simulink model "gm_CustArchitecture_vnl"  (R2020a)
settings: Solver=FixedStepDiscrete  StartTime=0.0  StopTime=840000  RelTol=1e-3
libraries: simulink x92, hdlsllib x56, IIT_Genoa_Intan_HDL_blocks x7
(part 1 of 3)
settings Model: FPTRunName=FPA_Reference  PacingRate=40  Creator=BuccelliLab  LastModifiedBy=diflo
settings SolverCC: AutoInsertRateTranBlk=on  MinimalZcImpactIntegration=on
settings DataIOCC: LimitDataPoints=on  SaveOutput=off  SaveTime=off  ReturnWorkspaceOutputs=off
settings OptimizationCC: BlockReduction=off  ConditionallyExecuteInputs=off  DefaultParameterBehavior=Inlined  LifeSpan=inf
settings DebuggingCC: SignalRangeChecking=warning  ReadBeforeWriteMsg=DisableAll  WriteAfterWriteMsg=DisableAll  WriteAfterReadMsg=DisableAll  AlgebraicLoopMsg=error  InheritedTsInSrcMsg=none  MultiTaskDSMMsg=none  SingleTaskRateTransMsg=error  ParameterDowncastMsg=warning  ParameterOverflowMsg=warning  AllowSymbolicDim=off  StrictBusMsg=ErrorOnBusTreatedAsVector  SFUnexpectedBacktrackingDiag=warning  SFNoUnconditionalDefaultTransitionDiag=warning  SFExecutionAtInitializationDiag=none  ArithmeticOperatorsInVariantConditions=warning
settings HardwareCC: ProdBitPerPointer=32  ProdBitPerSizeT=32  ProdBitPerPtrDiffT=32  ProdLargestAtomicFloat=None  ProdIntDivRoundTo=Undefined  ProdEndianess=Unspecified  ProdWordSize=32  ProdHWDeviceType=ASIC/FPGA->ASIC/FPGA  TargetBitPerPointer=64  TargetBitPerSizeT=64  TargetBitPerPtrDiffT=64  TargetLongLongMode=on  TargetIntDivRoundTo=Zero  TargetEndianess=LittleEndian  TargetWordSize=64  TargetHWDeviceType=Custom Processor->MATLAB Host Computer  ProdEqTarget=off
settings ModelReferenceCC: UpdateModelReferenceTargets=IfOutOfDate
settings SFSimCC: SFSimEcho=off  SimUseLocalCustomCode=off  CustomCodeUndefinedFunction=UseInterfaceOnly
settings RTWCC: RTWUseLocalCustomCode=off
settings CodeAppCC: StateflowObjectComments=on
settings GRTTargetCC: TargetLangStandard=C89/C90 (ANSI)
settings ConfigComp: CovScope=ReferencedModels  CovMetricSettings=dw  CovHtmlReporting=on  CovSaveCumulativeToWorkspaceVar=on  CovSaveSingleToWorkspaceVar=on  CovExternalEMLEnable=off  CovSFcnEnable=off

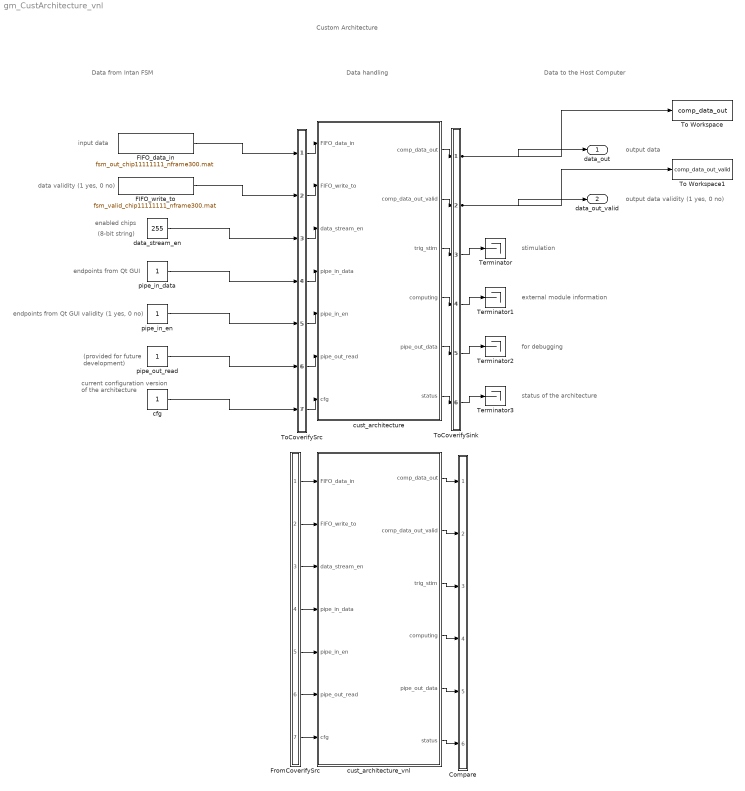
== system gm_CustArchitecture_vnl ==
  note: Data handling
  note: Custom Architecture
  note: output data validity (1 yes, 0 no)
  note: endpoints from Qt GUI
  note: (8-bit string)
  note: enabled chips
  note: data validity (1 yes, 0 no)
  note: input data
  note: endpoints from Qt GUI validity (1 yes, 0 no)
  note: (provided for future
      | development)
  note: current configuration
      | version of the
      | architecture
  note: output data
  note: Data to the Host Computer
  note: stimulation
  note: external module information
  note: for debugging
  note: status of the architecture
  note: Data from Intan FSM
  Compare : Subsystem
      mask Display: disp('')
  FIFO_data_in : FromFile  FileName=fsm_out_chip11111111_nframe300.mat  OutDataTypeStr=uint16  SampleTime=1  ExtrapolationBeforeFirstDataPoint=Hold first value  InterpolationWithinTimeRange=Zero order hold  ExtrapolationAfterLastDataPoint=Hold last value
  FIFO_write_to : FromFile  FileName=fsm_valid_chip11111111_nframe300.mat  OutDataTypeStr=boolean  SampleTime=1
  FromCoverifySrc : Subsystem
      mask Display: disp('')
  Terminator{,1..3} (4 alike) : Terminator
  To Workspace : ToWorkspace  VariableName=comp_data_out  SaveFormat=Timeseries  SampleTime=-1
  To Workspace1 : ToWorkspace  VariableName=comp_data_out_valid  SaveFormat=Timeseries  SampleTime=-1
  ToCoverifySink : Subsystem
      mask Display: disp('')
  ToCoverifySrc : Subsystem
      mask Display: disp('')
  cfg : Constant  OutDataTypeStr=uint16  SampleTime=-1
  cust_architecture : Subsystem
  cust_architecture_vnl : Subsystem
  data_stream_en : Constant  Value=255  OutDataTypeStr=uint8  SampleTime=-1
  pipe_in_data : Constant  OutDataTypeStr=uint16  SampleTime=-1
  pipe_in_en : Constant  OutDataTypeStr=boolean  SampleTime=-1
  pipe_out_read : Constant  OutDataTypeStr=boolean  SampleTime=-1
  data_out : Outport  VectorParamsAs1DForOutWhenUnconnected=off
  data_out_valid : Outport  Port=2  VectorParamsAs1DForOutWhenUnconnected=off
  wires:
  ToCoverifySrc/1(out1) -> cust_architecture/1(FIFO_data_in)
  ToCoverifySrc/2(out2) -> cust_architecture/2(FIFO_write_to)
  ToCoverifySrc/3(out3) -> cust_architecture/3(data_stream_en)
  ToCoverifySrc/4(out4) -> cust_architecture/4(pipe_in_data)
  ToCoverifySrc/5(out5) -> cust_architecture/5(pipe_in_en)
  ToCoverifySrc/6(out6) -> cust_architecture/6(pipe_out_read)
  ToCoverifySrc/7(out7) -> cust_architecture/7(cfg)
  cust_architecture/1(comp_data_out) -> ToCoverifySink/1(in1)
  cust_architecture/2(comp_data_out_valid) -> ToCoverifySink/2(in2)
  cust_architecture/3(trig_stim) -> ToCoverifySink/3(in3)
  cust_architecture/4(computing) -> ToCoverifySink/4(in4)
  cust_architecture/5(pipe_out_data) -> ToCoverifySink/5(in5)
  cust_architecture/6(status) -> ToCoverifySink/6(in6)
  FIFO_data_in/1 -> ToCoverifySrc/1(in1)
  FIFO_write_to/1 -> ToCoverifySrc/2(in2)
  data_stream_en/1 -> ToCoverifySrc/3(in3)
  pipe_in_data/1 -> ToCoverifySrc/4(in4)
  pipe_in_en/1 -> ToCoverifySrc/5(in5)
  pipe_out_read/1 -> ToCoverifySrc/6(in6)
  cfg/1 -> ToCoverifySrc/7(in7)
  ToCoverifySink/1(out1) -> data_out/1, To Workspace/1
  ToCoverifySink/2(out2) -> data_out_valid/1, To Workspace1/1
  ToCoverifySink/3(out3) -> Terminator/1
  ToCoverifySink/4(out4) -> Terminator1/1
  ToCoverifySink/5(out5) -> Terminator2/1
  ToCoverifySink/6(out6) -> Terminator3/1
  FromCoverifySrc/1(out1) -> cust_architecture_vnl/1(FIFO_data_in)
  FromCoverifySrc/2(out2) -> cust_architecture_vnl/2(FIFO_write_to)
  FromCoverifySrc/3(out3) -> cust_architecture_vnl/3(data_stream_en)
  FromCoverifySrc/4(out4) -> cust_architecture_vnl/4(pipe_in_data)
  FromCoverifySrc/5(out5) -> cust_architecture_vnl/5(pipe_in_en)
  FromCoverifySrc/6(out6) -> cust_architecture_vnl/6(pipe_out_read)
  FromCoverifySrc/7(out7) -> cust_architecture_vnl/7(cfg)
  cust_architecture_vnl/1(comp_data_out) -> Compare/1(in1)
  cust_architecture_vnl/2(comp_data_out_valid) -> Compare/2(in2)
  cust_architecture_vnl/3(trig_stim) -> Compare/3(in3)
  cust_architecture_vnl/4(computing) -> Compare/4(in4)
  cust_architecture_vnl/5(pipe_out_data) -> Compare/5(in5)
  cust_architecture_vnl/6(status) -> Compare/6(in6)

== system gm_CustArchitecture_vnl/Compare ==
  in1 : Inport
  in2 : Inport  Port=2
  in3 : Inport  Port=3
  in4 : Inport  Port=4
  in5 : Inport  Port=5
  in6 : Inport  Port=6
  Assert_comp_data_out : Subsystem
  Assert_comp_data_out_valid : Subsystem
  Assert_computing : Subsystem
  Assert_pipe_out_data : Subsystem
  Assert_status : Subsystem
  Assert_trig_stim : Subsystem
  CleanupScopes : Subsystem
      settings: OpenFcn=|
      | blkName = gcb; %self block
      | idx = regexp(blkName, '/CleanupScopes$', 'once');
      | blkParent = blkName(1:idx-1);
      | blks=find_system(blkParent, 'LookUnderMasks', 'all','blocktype', 'Scope');
      | for itr = 1:length(blks)
      | 	 hScopeCfg = get_param(blks{itr},'ScopeConfiguration');
      | 	 hScopeCfg.Visible = ~ hScopeCfg.Visible;
      | end
      | drawnow;
      mask Display: fprintf(message('hdlcoder:cosim:vnl_dblclick').getString());
  Enable : Subsystem
      settings: OpenFcn=|
      | blkName = gcb;
      | idx = regexp(blkName, '/Enable$', 'once');
      | blkParent = blkName(1:idx-1);
      | blks=find_system(blkParent, 'LookUnderMasks', 'all','blocktype', 'Assertion');
      | e = get_param(blks{1}, 'Enabled');
      | if strcmp(e, 'on'), f= 'off';, else, f = 'on';, end
      | for ii=1:length(blks), set_param(blks{ii}, 'Enabled', f);, end
      | set_param(gcb, 'MaskDisplay',['fprintf(message(''hdlcoder:cosim:vnl_dblclick_assertions'',','''',upper(e),'''',').getString())']);
      mask Display: fprintf(message('hdlcoder:cosim:vnl_dblclick_assertions','OFF').getString());
  wires:
  in1/1 -> Assert_comp_data_out/1(cosim)
  [out1] -> Assert_comp_data_out/2(dut)
  in2/1 -> Assert_comp_data_out_valid/1(cosim)
  [out2] -> Assert_comp_data_out_valid/2(dut)
  in3/1 -> Assert_trig_stim/1(cosim)
  [out3] -> Assert_trig_stim/2(dut)
  in4/1 -> Assert_computing/1(cosim)
  [out4] -> Assert_computing/2(dut)
  in5/1 -> Assert_pipe_out_data/1(cosim)
  [out5] -> Assert_pipe_out_data/2(dut)
  in6/1 -> Assert_status/1(cosim)
  [out6] -> Assert_status/2(dut)

== system gm_CustArchitecture_vnl/FromCoverifySrc ==
  out1 : Outport
  out2 : Outport  Port=2
  out3 : Outport  Port=3
  out4 : Outport  Port=4
  out5 : Outport  Port=5
  out6 : Outport  Port=6
  out7 : Outport  Port=7
  wires:
  [in1] -> out1/1
  [in2] -> out2/1
  [in3] -> out3/1
  [in4] -> out4/1
  [in5] -> out5/1
  [in6] -> out6/1
  [in7] -> out7/1

== system gm_CustArchitecture_vnl/ToCoverifySink ==
  in1 : Inport
  in2 : Inport  Port=2
  in3 : Inport  Port=3
  in4 : Inport  Port=4
  in5 : Inport  Port=5
  in6 : Inport  Port=6
  out1 : Outport
  out2 : Outport  Port=2
  out3 : Outport  Port=3
  out4 : Outport  Port=4
  out5 : Outport  Port=5
  out6 : Outport  Port=6
  tag scope: out1=global, out2=global, out3=global, out4=global, out5=global, out6=global
  wires:
  in1/1 -> out1/1, [out1]
  in2/1 -> out2/1, [out2]
  in3/1 -> out3/1, [out3]
  in4/1 -> out4/1, [out4]
  in5/1 -> out5/1, [out5]
  in6/1 -> out6/1, [out6]

== system gm_CustArchitecture_vnl/ToCoverifySrc ==
  in1 : Inport
  in2 : Inport  Port=2
  in3 : Inport  Port=3
  in4 : Inport  Port=4
  in5 : Inport  Port=5
  in6 : Inport  Port=6
  in7 : Inport  Port=7
  out1 : Outport
  out2 : Outport  Port=2
  out3 : Outport  Port=3
  out4 : Outport  Port=4
  out5 : Outport  Port=5
  out6 : Outport  Port=6
  out7 : Outport  Port=7
  tag scope: in1=global, in2=global, in3=global, in4=global, in5=global, in6=global, in7=global
  wires:
  in1/1 -> out1/1, [in1]
  in2/1 -> out2/1, [in2]
  in3/1 -> out3/1, [in3]
  in4/1 -> out4/1, [in4]
  in5/1 -> out5/1, [in5]
  in6/1 -> out6/1, [in6]
  in7/1 -> out7/1, [in7]

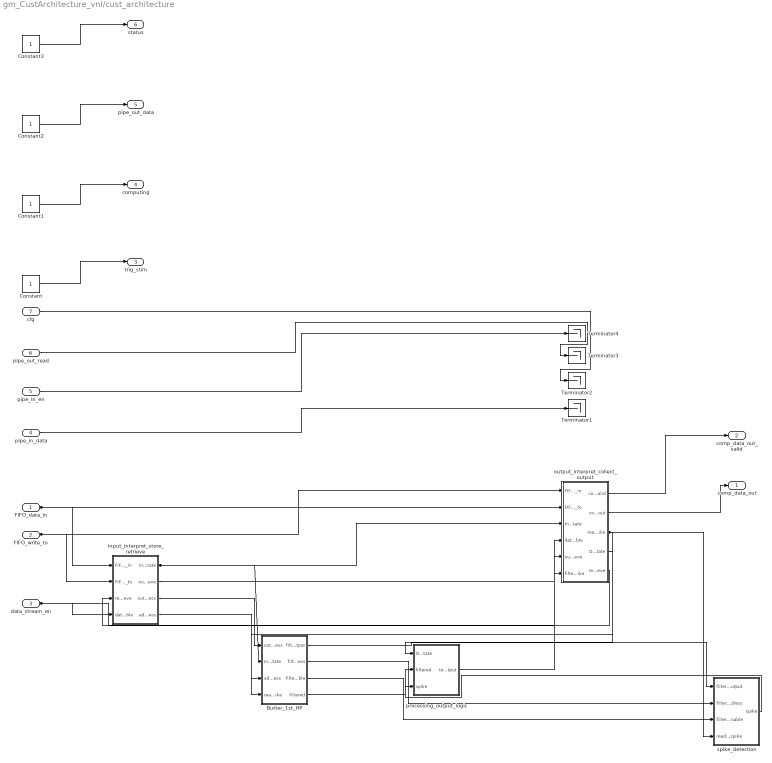
== system gm_CustArchitecture_vnl/cust_architecture ==
  FIFO_data_in : Inport  OutDataTypeStr=uint16  PortDimensions=1  SampleTime=1
  FIFO_write_to : Inport  Port=2  OutDataTypeStr=boolean  PortDimensions=1  SampleTime=1
  data_stream_en : Inport  Port=3  OutDataTypeStr=uint8  PortDimensions=1  SampleTime=1
  pipe_in_data : Inport  Port=4  OutDataTypeStr=uint16  PortDimensions=1  SampleTime=1
  pipe_in_en : Inport  Port=5  OutDataTypeStr=boolean  PortDimensions=1  SampleTime=1
  pipe_out_read : Inport  Port=6  OutDataTypeStr=boolean  PortDimensions=1  SampleTime=1
  cfg : Inport  Port=7  OutDataTypeStr=uint16  PortDimensions=1  SampleTime=1
  Butter_1st_HP : Subsystem  mask{s1=double(0.9695312529087462), a21=double(-0.9390625058174924)}
      mask Display:
      | color('white'); port_label('input',1,'output_data_to_process')
      | color('white'); port_label('input',2,'InputState')
      | color('white'); port_label('input',3,'address_output_data_to_process')
      | color('white'); port_label('input',4,'read_filter_output_or_spike')
      | color('white'); port_label('output',1,'filter_output')
      | color('white'); port_label('output',2,'filter_writing_address')
      | color('white'); port_label('output',3,'filter_writing_enable')
      | color('white'); port_label('output',4,'filtered')
  Constant : Constant  OutDataTypeStr=uint8  SampleTime=1
  Constant1 : Constant  OutDataTypeStr=boolean  SampleTime=1
  Constant2 : Constant  OutDataTypeStr=uint16  SampleTime=1
  Constant3 : Constant  OutDataTypeStr=uint16  SampleTime=1
  Terminator{1..4} (4 alike) : Terminator
  input_interpret_store_retrieve : Subsystem
  output_interpret_collect_output : Subsystem
  processing_output_logic : Subsystem
  spike_detection : Subsystem
  comp_data_out : Outport  VectorParamsAs1DForOutWhenUnconnected=off
  comp_data_out_valid : Outport  Port=2  OutDataTypeStr=boolean  VectorParamsAs1DForOutWhenUnconnected=off
  trig_stim : Outport  Port=3  VectorParamsAs1DForOutWhenUnconnected=off
  computing : Outport  Port=4  VectorParamsAs1DForOutWhenUnconnected=off
  pipe_out_data : Outport  Port=5  VectorParamsAs1DForOutWhenUnconnected=off
  status : Outport  Port=6  VectorParamsAs1DForOutWhenUnconnected=off
  wires:
  spike_detection/1(spike) -> processing_output_logic/3(spike)
  processing_output_logic/1(to_output_interpret_collect_output) -> output_interpret_collect_output/6(filter_output_or_spike)
  output_interpret_collect_output/5(read_output_data_input_interpret_store_retrieve) -> input_interpret_store_retrieve/3(read_output_data_input_interpret_store_retrieve)
  output_interpret_collect_output/4(OutputState) -> processing_output_logic/1(OutputState)
  output_interpret_collect_output/3(read_filter_output_or_spike) -> Butter_1st_HP/4(read_filter_output_or_spike), spike_detection/4(read_filter_output_or_spike)
  output_interpret_collect_output/2(comp_data_out) -> comp_data_out/1
  output_interpret_collect_output/1(comp_data_out_valid) -> comp_data_out_valid/1
  input_interpret_store_retrieve/4(address_output_data_to_process) -> Butter_1st_HP/3(address_output_data_to_process)
  input_interpret_store_retrieve/3(output_data_to_process) -> Butter_1st_HP/1(output_data_to_process)
  input_interpret_store_retrieve/2(output_data_input_interpret_store_retrieve) -> output_interpret_collect_output/5(output_data_input_interpret_store_retrieve)
  input_interpret_store_retrieve/1(InputState) -> output_interpret_collect_output/3(InputState), Butter_1st_HP/2(InputState)
  Constant3/1 -> status/1
  Constant2/1 -> pipe_out_data/1
  Constant1/1 -> computing/1
  Constant/1 -> trig_stim/1
  Butter_1st_HP/4(filtered) -> processing_output_logic/2(filtered)
  Butter_1st_HP/3(filter_writing_enable) -> spike_detection/3(filter_writing_enable)
  Butter_1st_HP/2(filter_writing_address) -> spike_detection/2(filter_writing_address)
  Butter_1st_HP/1(filter_output) -> spike_detection/1(filter_output)
  cfg/1 -> Terminator2/1
  pipe_out_read/1 -> Terminator3/1
  pipe_in_en/1 -> Terminator4/1
  pipe_in_data/1 -> Terminator1/1
  data_stream_en/1 -> input_interpret_store_retrieve/4(data_stream_enable), output_interpret_collect_output/4(data_stream_enable)
  FIFO_write_to/1 -> output_interpret_collect_output/2(FIFO_write_to), input_interpret_store_retrieve/2(FIFO_write_to)
  FIFO_data_in/1 -> output_interpret_collect_output/1(FIFO_data_in), input_interpret_store_retrieve/1(FIFO_data_in)

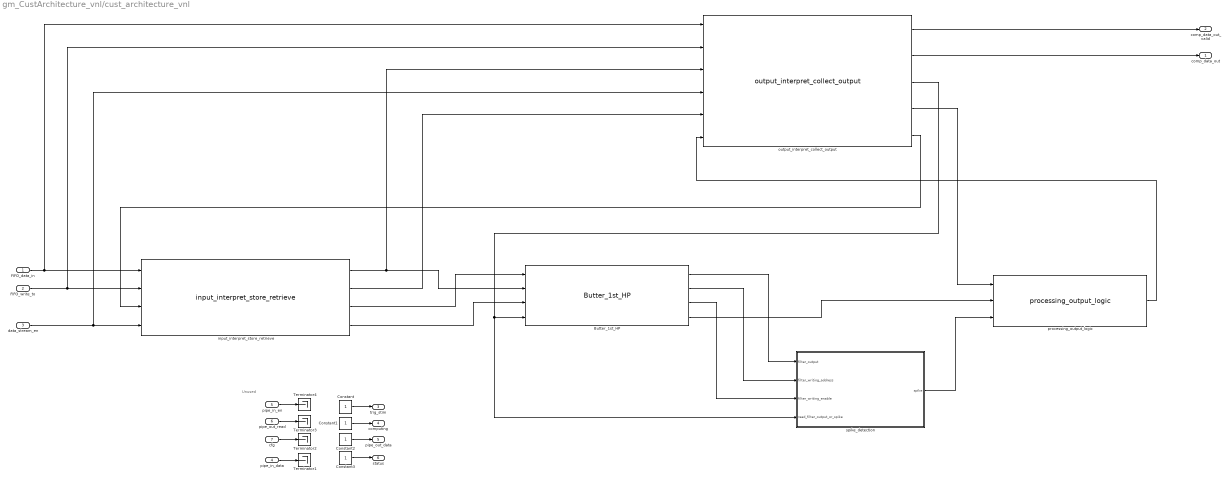
== system gm_CustArchitecture_vnl/cust_architecture_vnl ==
  note: Unused
  FIFO_data_in : Inport
  FIFO_write_to : Inport  Port=2
  data_stream_en : Inport  Port=3
  pipe_in_data : Inport  Port=4
  pipe_in_en : Inport  Port=5
  pipe_out_read : Inport  Port=6
  cfg : Inport  Port=7
  Butter_1st_HP : IIT_Genoa_Intan_HDL_blocks/Filters/Butter_1st_HP  s1=0.969531252908746199  a21=-0.939062505817492399
      settings: SourceProductName=IIT Genoa Intan HDL blocks
  Constant : Constant  OutDataTypeStr=uint8  SampleTime=-1
  Constant1 : Constant  OutDataTypeStr=boolean  SampleTime=-1
  Constant2 : Constant  OutDataTypeStr=uint16  SampleTime=-1
  Constant3 : Constant  OutDataTypeStr=uint16  SampleTime=-1
  Terminator{1..4} (4 alike) : Terminator
  input_interpret_store_retrieve : IIT_Genoa_Intan_HDL_blocks/Encoding//Decoding/input_interpret_store_retrieve
      settings: SourceProductName=IIT Genoa Intan HDL blocks
  output_interpret_collect_output : IIT_Genoa_Intan_HDL_blocks/Encoding//Decoding/output_interpret_collect_output
      settings: SourceProductName=IIT Genoa Intan HDL blocks
  processing_output_logic : IIT_Genoa_Intan_HDL_blocks/Encoding//Decoding/processing_output_logic
      settings: SourceProductName=IIT Genoa Intan HDL blocks
  spike_detection : Subsystem
  comp_data_out : Outport  VectorParamsAs1DForOutWhenUnconnected=off
  comp_data_out_valid : Outport  Port=2  OutDataTypeStr=boolean  VectorParamsAs1DForOutWhenUnconnected=off
  trig_stim : Outport  Port=3  VectorParamsAs1DForOutWhenUnconnected=off
  computing : Outport  Port=4  VectorParamsAs1DForOutWhenUnconnected=off
  pipe_out_data : Outport  Port=5  VectorParamsAs1DForOutWhenUnconnected=off
  status : Outport  Port=6  VectorParamsAs1DForOutWhenUnconnected=off
  wires:
  input_interpret_store_retrieve/4 -> Butter_1st_HP/3
  input_interpret_store_retrieve/3 -> Butter_1st_HP/1
  spike_detection/1(spike) -> processing_output_logic/3
  Butter_1st_HP/3 -> spike_detection/3(filter_writing_enable)
  Butter_1st_HP/2 -> spike_detection/2(filter_writing_address)
  Butter_1st_HP/1 -> spike_detection/1(filter_output)
  processing_output_logic/1 -> output_interpret_collect_output/6
  input_interpret_store_retrieve/1 -> output_interpret_collect_output/3, Butter_1st_HP/2
  input_interpret_store_retrieve/2 -> output_interpret_collect_output/5
  Butter_1st_HP/4 -> processing_output_logic/2
  output_interpret_collect_output/3 -> Butter_1st_HP/4, spike_detection/4(read_filter_output_or_spike)
  output_interpret_collect_output/4 -> processing_output_logic/1
  output_interpret_collect_output/5 -> input_interpret_store_retrieve/3
  output_interpret_collect_output/2 -> comp_data_out/1
  output_interpret_collect_output/1 -> comp_data_out_valid/1
  pipe_in_data/1 -> Terminator1/1
  data_stream_en/1 -> input_interpret_store_retrieve/4, output_interpret_collect_output/4
  FIFO_write_to/1 -> output_interpret_collect_output/2, input_interpret_store_retrieve/2
  FIFO_data_in/1 -> output_interpret_collect_output/1, input_interpret_store_retrieve/1
  pipe_in_en/1 -> Terminator4/1
  pipe_out_read/1 -> Terminator3/1
  cfg/1 -> Terminator2/1
  Constant3/1 -> status/1
  Constant2/1 -> pipe_out_data/1
  Constant1/1 -> computing/1
  Constant/1 -> trig_stim/1

== system gm_CustArchitecture_vnl/Compare/Assert_comp_data_out ==
  cosim : Inport
  dut : Inport  Port=2
  AssertEq : Assertion  StopWhenAssertionFail=off
  Compare To Zero : simulink/Logic and Bit Operations/Compare To Zero  relop===  OutDataTypeStr=boolean
  Relational Operator : RelationalOperator  Operator===  OutDataTypeStr=boolean  RndMeth=Nearest
  compare: comp_data_out : Scope  NumInputPorts=3
  wires:
  Compare To Zero/1 -> compare: comp_data_out/3  "err"
  Relational Operator/1 -> Compare To Zero/1, AssertEq/1
  cosim/1 -> compare: comp_data_out/1, Relational Operator/1  "cosim"
  dut/1 -> compare: comp_data_out/2, Relational Operator/2  "dut ref"

== system gm_CustArchitecture_vnl/Compare/Assert_comp_data_out_valid ==
  cosim : Inport
  dut : Inport  Port=2
  AssertEq : Assertion  StopWhenAssertionFail=off
  Compare To Zero : simulink/Logic and Bit Operations/Compare To Zero  relop===  OutDataTypeStr=boolean
  Relational Operator : RelationalOperator  Operator===  OutDataTypeStr=boolean  RndMeth=Nearest
  compare: comp_data_out_valid : Scope  NumInputPorts=3
  wires:
  Compare To Zero/1 -> compare: comp_data_out_valid/3  "err"
  Relational Operator/1 -> Compare To Zero/1, AssertEq/1
  cosim/1 -> compare: comp_data_out_valid/1, Relational Operator/1  "cosim"
  dut/1 -> compare: comp_data_out_valid/2, Relational Operator/2  "dut ref"

== system gm_CustArchitecture_vnl/Compare/Assert_computing ==
  cosim : Inport
  dut : Inport  Port=2
  AssertEq : Assertion  StopWhenAssertionFail=off
  Compare To Zero : simulink/Logic and Bit Operations/Compare To Zero  relop===  OutDataTypeStr=boolean
  Relational Operator : RelationalOperator  Operator===  OutDataTypeStr=boolean  RndMeth=Nearest
  compare: computing : Scope  NumInputPorts=3
  wires:
  Compare To Zero/1 -> compare: computing/3  "err"
  Relational Operator/1 -> Compare To Zero/1, AssertEq/1
  cosim/1 -> compare: computing/1, Relational Operator/1  "cosim"
  dut/1 -> compare: computing/2, Relational Operator/2  "dut ref"

== system gm_CustArchitecture_vnl/Compare/Assert_pipe_out_data ==
  cosim : Inport
  dut : Inport  Port=2
  AssertEq : Assertion  StopWhenAssertionFail=off
  Compare To Zero : simulink/Logic and Bit Operations/Compare To Zero  relop===  OutDataTypeStr=boolean
  Relational Operator : RelationalOperator  Operator===  OutDataTypeStr=boolean  RndMeth=Nearest
  compare: pipe_out_data : Scope  NumInputPorts=3
  wires:
  Compare To Zero/1 -> compare: pipe_out_data/3  "err"
  Relational Operator/1 -> Compare To Zero/1, AssertEq/1
  cosim/1 -> compare: pipe_out_data/1, Relational Operator/1  "cosim"
  dut/1 -> compare: pipe_out_data/2, Relational Operator/2  "dut ref"

== system gm_CustArchitecture_vnl/Compare/Assert_status ==
  cosim : Inport
  dut : Inport  Port=2
  AssertEq : Assertion  StopWhenAssertionFail=off
  Compare To Zero : simulink/Logic and Bit Operations/Compare To Zero  relop===  OutDataTypeStr=boolean
  Relational Operator : RelationalOperator  Operator===  OutDataTypeStr=boolean  RndMeth=Nearest
  compare: status : Scope  NumInputPorts=3
  wires:
  Compare To Zero/1 -> compare: status/3  "err"
  Relational Operator/1 -> Compare To Zero/1, AssertEq/1
  cosim/1 -> compare: status/1, Relational Operator/1  "cosim"
  dut/1 -> compare: status/2, Relational Operator/2  "dut ref"

== system gm_CustArchitecture_vnl/Compare/Assert_trig_stim ==
  cosim : Inport
  dut : Inport  Port=2
  AssertEq : Assertion  StopWhenAssertionFail=off
  Compare To Zero : simulink/Logic and Bit Operations/Compare To Zero  relop===  OutDataTypeStr=boolean
  Relational Operator : RelationalOperator  Operator===  OutDataTypeStr=boolean  RndMeth=Nearest
  compare: trig_stim : Scope  NumInputPorts=3
  wires:
  Compare To Zero/1 -> compare: trig_stim/3  "err"
  Relational Operator/1 -> Compare To Zero/1, AssertEq/1
  cosim/1 -> compare: trig_stim/1, Relational Operator/1  "cosim"
  dut/1 -> compare: trig_stim/2, Relational Operator/2  "dut ref"

== system gm_CustArchitecture_vnl/Compare/CleanupScopes ==

== system gm_CustArchitecture_vnl/Compare/Enable ==

== system gm_CustArchitecture_vnl/cust_architecture/Butter_1st_HP ==
  output_data_to_process : Inport  OutDataTypeStr=uint16  SampleTime=1
  InputState : Inport  Port=2  OutDataTypeStr=uint8  SampleTime=1
  address_output_data_to_process : Inport  Port=3  OutDataTypeStr=fixdt(0, 9, 0)  SampleTime=1
  read_filter_output_or_spike : Inport  Port=4  OutDataTypeStr=fixdt(0, 9, 0)  SampleTime=1
  ProcessedData_storage : hdlsllib/HDL RAMs/Dual Port RAM  ram_size=9
      settings: SourceProductBaseCode=SL
  Subsystem : Subsystem
  Terminator1 : Terminator
  filter_output : Outport
  filter_writing_address : Outport  Port=2
  filter_writing_enable : Outport  Port=3
  filtered : Outport  Port=4
  wires:
  Subsystem/3(filter_writing_enable) -> ProcessedData_storage/3, filter_writing_enable/1
  Subsystem/2(filter_writing_address) -> ProcessedData_storage/2, filter_writing_address/1
  Subsystem/1(filter_output) -> ProcessedData_storage/1, filter_output/1
  ProcessedData_storage/2 -> filtered/1
  ProcessedData_storage/1 -> Terminator1/1
  read_filter_output_or_spike/1 -> ProcessedData_storage/4
  address_output_data_to_process/1 -> Subsystem/3(address_output_data_to_process)
  InputState/1 -> Subsystem/2(InputState)
  output_data_to_process/1 -> Subsystem/1(output_data_to_process)

== system gm_CustArchitecture_vnl/cust_architecture/input_interpret_store_retrieve ==
  note: address sent for processing
  note: data sent for processing
  note: data sent to Output
  FIFO_data_in : Inport  OutDataTypeStr=uint16  SampleTime=1
  FIFO_write_to : Inport  Port=2  OutDataTypeStr=boolean  SampleTime=1
  read_output_data_input_interpret_store_retrieve : Inport  Port=3  OutDataTypeStr=fixdt(0, 9, 0)  SampleTime=1
  data_stream_enable : Inport  Port=4  OutDataTypeStr=uint8  SampleTime=1
  InputStateMachine : Subsystem
  Interpret_to_RAM_input : Subsystem
  store_and_retrieve_input : Subsystem
  InputState : Outport
  output_data_input_interpret_store_retrieve : Outport  Port=2
  output_data_to_process : Outport  Port=3
  address_output_data_to_process : Outport  Port=4
  wires:
  store_and_retrieve_input/3(read_from_porcessing_addr) -> address_output_data_to_process/1
  store_and_retrieve_input/2(current_value) -> output_data_to_process/1
  store_and_retrieve_input/1(read_from_storage_value) -> output_data_input_interpret_store_retrieve/1
  Interpret_to_RAM_input/5(wr_en) -> store_and_retrieve_input/4(wr_en)
  Interpret_to_RAM_input/4(write address) -> store_and_retrieve_input/3(wr_address)
  Interpret_to_RAM_input/3(wr_din) -> store_and_retrieve_input/2(wr_din)
  Interpret_to_RAM_input/2(inc_source_device) -> InputStateMachine/4(inc_source_device_MSB)
  Interpret_to_RAM_input/1(device_output) -> InputStateMachine/3(channel_0_19)
  InputStateMachine/1(InputState) -> store_and_retrieve_input/5(InputState), InputState/1, Interpret_to_RAM_input/3(InputState)
  data_stream_enable/1 -> Interpret_to_RAM_input/4(data_stream_enable)
  read_output_data_input_interpret_store_retrieve/1 -> store_and_retrieve_input/1(read address)
  FIFO_write_to/1 -> Interpret_to_RAM_input/2(FIFO_write_to), InputStateMachine/2(FIFO_write_to)
  FIFO_data_in/1 -> Interpret_to_RAM_input/1(FIFO_data_in), InputStateMachine/1(FIFO_data_in)

== system gm_CustArchitecture_vnl/cust_architecture/output_interpret_collect_output ==
  FIFO_data_in : Inport  OutDataTypeStr=uint16  SampleTime=1
  FIFO_write_to : Inport  Port=2  OutDataTypeStr=boolean  SampleTime=1
  InputState : Inport  Port=3  OutDataTypeStr=uint8  SampleTime=1
  data_stream_enable : Inport  Port=4  OutDataTypeStr=uint8  SampleTime=1
  output_data_input_interpret_store_retrieve : Inport  Port=5  OutDataTypeStr=uint16  SampleTime=1
  filter_output_or_spike : Inport  Port=6  OutDataTypeStr=uint16  SampleTime=1
  collect_output : Subsystem
  output_interpret : Subsystem
  comp_data_out_valid : Outport
  comp_data_out : Outport  Port=2
  read_filter_output_or_spike : Outport  Port=3
  OutputState : Outport  Port=4
  read_output_data_input_interpret_store_retrieve : Outport  Port=5
  wires:
  output_interpret/3(read_output_data_input_interpret_store_retrieve) -> read_output_data_input_interpret_store_retrieve/1, collect_output/6(rd_address)
  output_interpret/2(rd_enable) -> collect_output/5(rd_enable)
  output_interpret/1(OutputState) -> OutputState/1, collect_output/4(OutputState)
  collect_output/3(rd_address_bit_set_AC_during_DC) -> read_filter_output_or_spike/1
  collect_output/2(comp_data_out) -> comp_data_out/1
  collect_output/1(comp_data_out_valid) -> comp_data_out_valid/1
  filter_output_or_spike/1 -> collect_output/8(rd_dout)
  output_data_input_interpret_store_retrieve/1 -> collect_output/7(read_from_storage_value)
  data_stream_enable/1 -> output_interpret/1(data_stream_enable)
  InputState/1 -> output_interpret/2(InputState), collect_output/3(InputState)
  FIFO_write_to/1 -> collect_output/2(FIFO_write_to)
  FIFO_data_in/1 -> collect_output/1(FIFO_data_in)

== system gm_CustArchitecture_vnl/cust_architecture/processing_output_logic ==
  OutputState : Inport  OutDataTypeStr=uint8  SampleTime=1
  filtered : Inport  Port=2  OutDataTypeStr=uint16  SampleTime=1
  spike : Inport  Port=3  OutDataTypeStr=uint16  SampleTime=1
  Delay : Delay  DelayLength=double(1)  InitialCondition=0  SampleTime=1
  Switch : Switch  Criteria=u2 > Threshold  Threshold=double(6)  OutDataTypeStr=uint16  SampleTime=1
  to_output_interpret_collect_output : Outport
  wires:
  Switch/1 -> to_output_interpret_collect_output/1
  Delay/1 -> Switch/2
  spike/1 -> Switch/3
  filtered/1 -> Switch/1
  OutputState/1 -> Delay/1

== system gm_CustArchitecture_vnl/cust_architecture/spike_detection ==
  filter_output : Inport  OutDataTypeStr=uint16  PortDimensions=1  SampleTime=1
  filter_writing_address : Inport  Port=2  OutDataTypeStr=fixdt(0, 9, 0)  PortDimensions=1  SampleTime=1
  filter_writing_enable : Inport  Port=3  OutDataTypeStr=boolean  PortDimensions=1  SampleTime=1
  read_filter_output_or_spike : Inport  Port=4  OutDataTypeStr=fixdt(0, 9, 0)  PortDimensions=1  SampleTime=1
  LocalMaxima : Subsystem  mask{th=double(0)}
      mask prompts: th "Threshold (µV)"
      mask Display:
      | color('white'); port_label('input',1,'filter_output')
      | color('white'); port_label('input',2,'filter_writing_enable')
      | color('white'); port_label('input',3,'filter_writing_address')
      | color('white'); port_label('output',1,'detection_check')
  refractory_period : Subsystem  mask{refractory=double(30)}
      mask prompts: refractory "Refractory period (samples)"
      mask Display:
      | color('white'); port_label('input',1,'filter_writing_enable')
      | color('white'); port_label('input',2,'spike_check')
      | color('white'); port_label('input',3,'filter_writing_address')
      | color('white'); port_label('input',4,'read_filter_output_or_spike')
      | color('white'); port_label('output',1,'refractory_check')
      | color('white'); port_label('output',2,'spike')
  spike_check : Subsystem
  spike : Outport
  wires:
  spike_check/1(spike_check) -> refractory_period/2(spike_check)
  refractory_period/2(spike) -> spike/1
  refractory_period/1(refractory_check) -> spike_check/2(refractory_check)
  LocalMaxima/1(detection_check) -> spike_check/1(detection_check)
  read_filter_output_or_spike/1 -> refractory_period/4(read_filter_output_or_spike)
  filter_writing_enable/1 -> LocalMaxima/2(filter_writing_enable), refractory_period/1(filter_writing_enable)
  filter_writing_address/1 -> LocalMaxima/3(filter_writing_address), refractory_period/3(filter_writing_address)
  filter_output/1 -> LocalMaxima/1(filter_output)

== system gm_CustArchitecture_vnl/cust_architecture_vnl/spike_detection ==
  filter_output : Inport
  filter_writing_address : Inport  Port=2
  filter_writing_enable : Inport  Port=3
  read_filter_output_or_spike : Inport  Port=4
  LocalMaxima : IIT_Genoa_Intan_HDL_blocks/Spike Detection/Sample Thresholding/LocalMaxima  th=0
      settings: SourceProductName=IIT Genoa Intan HDL blocks
  refractory_period : IIT_Genoa_Intan_HDL_blocks/Spike Detection/General/refractory_period  refractory=30
      settings: SourceProductName=IIT Genoa Intan HDL blocks
  spike_check : IIT_Genoa_Intan_HDL_blocks/Spike Detection/General/spike_check
      settings: SourceProductName=IIT Genoa Intan HDL blocks
  spike : Outport
  wires:
  refractory_period/2 -> spike/1
  read_filter_output_or_spike/1 -> refractory_period/4
  filter_output/1 -> LocalMaxima/1
  filter_writing_enable/1 -> LocalMaxima/2, refractory_period/1
  refractory_period/1 -> spike_check/2
  filter_writing_address/1 -> LocalMaxima/3, refractory_period/3
  LocalMaxima/1 -> spike_check/1
  spike_check/1 -> refractory_period/2

== system gm_CustArchitecture_vnl/cust_architecture/Butter_1st_HP/Subsystem ==
  output_data_to_process : Inport  OutDataTypeStr=uint16  PortDimensions=1  SampleTime=1
  InputState : Inport  Port=2  OutDataTypeStr=uint8  PortDimensions=1  SampleTime=1
  address_output_data_to_process : Inport  Port=3  OutDataTypeStr=fixdt(0, 9, 0)  PortDimensions=1  SampleTime=1
  Memory2 : Memory  InheritSampleTime=on
  Memory3 : Memory  InheritSampleTime=on
  Memory5 : Memory  InheritSampleTime=on
  PreviousData_storage : hdlsllib/HDL RAMs/Dual Port RAM  ram_size=9
      settings: SourceProductBaseCode=SL
  Terminator8 : Terminator
  input_state_AC : simulink/Logic and Bit Operations/Compare To Constant  relop===  const=7  OutDataTypeStr=boolean
  one_pole_IIR : Subsystem
  filter_output : Outport
  filter_writing_address : Outport  Port=2
  filter_writing_enable : Outport  Port=3
  wires:
  one_pole_IIR/2(new_previous_sample) -> PreviousData_storage/1
  one_pole_IIR/1(filter_output) -> filter_output/1
  input_state_AC/1 -> Memory2/1
  PreviousData_storage/2 -> one_pole_IIR/2(previous_sample)
  PreviousData_storage/1 -> Terminator8/1
  Memory5/1 -> PreviousData_storage/2, filter_writing_address/1
  Memory3/1 -> input_state_AC/1
  Memory2/1 -> PreviousData_storage/3, filter_writing_enable/1
  address_output_data_to_process/1 -> PreviousData_storage/4, Memory5/1
  InputState/1 -> Memory3/1
  output_data_to_process/1 -> one_pole_IIR/1(output_data_to_process)

== system gm_CustArchitecture_vnl/cust_architecture/input_interpret_store_retrieve/InputStateMachine ==
  FIFO_data_in : Inport  OutDataTypeStr=uint16  PortDimensions=1  SampleTime=1
  FIFO_write_to : Inport  Port=2  OutDataTypeStr=boolean  PortDimensions=1  SampleTime=1
  channel_0_19 : Inport  Port=3  OutDataTypeStr=uint8  PortDimensions=1  SampleTime=1
  inc_source_device_MSB : Inport  Port=4  OutDataTypeStr=boolean  PortDimensions=1  SampleTime=1
  IIT_Genoa_Intan_HDL_blocks_c3_InputStateMachine : Stateflow chart  TreatAsAtomicUnit=on
  InputState : Outport  VectorParamsAs1DForOutWhenUnconnected=off
  wires:
  IIT_Genoa_Intan_HDL_blocks_c3_InputStateMachine/1(InputState) -> InputState/1
  inc_source_device_MSB/1 -> IIT_Genoa_Intan_HDL_blocks_c3_InputStateMachine/4(inc_source_device_MSB)
  channel_0_19/1 -> IIT_Genoa_Intan_HDL_blocks_c3_InputStateMachine/3(channel_0_19)
  FIFO_write_to/1 -> IIT_Genoa_Intan_HDL_blocks_c3_InputStateMachine/2(FIFO_write_to)
  FIFO_data_in/1 -> IIT_Genoa_Intan_HDL_blocks_c3_InputStateMachine/1(FIFO_data_in)

== system gm_CustArchitecture_vnl/cust_architecture/input_interpret_store_retrieve/Interpret_to_RAM_input ==
  FIFO_data_in : Inport  OutDataTypeStr=uint16  PortDimensions=1  SampleTime=1
  FIFO_write_to : Inport  Port=2  OutDataTypeStr=boolean  PortDimensions=1  SampleTime=1
  InputState : Inport  Port=3  OutDataTypeStr=uint8  PortDimensions=1  SampleTime=1
  data_stream_enable : Inport  Port=4  OutDataTypeStr=uint8  PortDimensions=1  SampleTime=1
  RAM address definition : Subsystem
  interpret incoming data : Subsystem
  device_output : Outport
  inc_source_device : Outport  Port=2
  wr_din : Outport  Port=3
  write address : Outport  Port=4
  wr_en : Outport  Port=5
  wires:
  interpret incoming data/5(converter_cnt) -> RAM address definition/5(converter_cnt)
  interpret incoming data/4(source_channel_0_159) -> RAM address definition/3(source_channel_0_159)
  interpret incoming data/3(device_output) -> device_output/1
  interpret incoming data/2(inc_source_device) -> inc_source_device/1
  interpret incoming data/1(source_device) -> RAM address definition/4(source_device)
  RAM address definition/3(write_enable_6to15) -> wr_en/1
  RAM address definition/2(wr_addr) -> write address/1
  RAM address definition/1(wr_din) -> wr_din/1
  data_stream_enable/1 -> interpret incoming data/3(data_stream_enable)
  InputState/1 -> RAM address definition/2(InputState), interpret incoming data/2(InputState)
  FIFO_write_to/1 -> RAM address definition/6(write_to), interpret incoming data/1(FIFO_write_to)
  FIFO_data_in/1 -> RAM address definition/1(DataIn)

== system gm_CustArchitecture_vnl/cust_architecture/input_interpret_store_retrieve/store_and_retrieve_input ==
  note: writing address
  note: address sent for processing
  note: current data
  note: data sent for processing
  note: data sent to Output
  note: current data
  read address : Inport  OutDataTypeStr=fixdt(0, 9, 0)  PortDimensions=1  SampleTime=1
  wr_din : Inport  Port=2  OutDataTypeStr=uint16  PortDimensions=1  SampleTime=1
  wr_address : Inport  Port=3  OutDataTypeStr=fixdt(0, 9, 0)  PortDimensions=1  SampleTime=1
  wr_en : Inport  Port=4  OutDataTypeStr=boolean  PortDimensions=1  SampleTime=1
  InputState : Inport  Port=5  OutDataTypeStr=uint8  PortDimensions=1  SampleTime=1
  Compare To Constant : simulink/Logic and Bit Operations/Compare To Constant  relop===  const="fi(0,0,8,0,\"hex\",\"07\")"  OutDataTypeStr=boolean
  Delay1 : Delay  DelayLength=double(1)  InitialCondition=0  SampleTime=1
  Terminator : Terminator
  Terminator6 : Terminator
  input_storage : hdlsllib/HDL RAMs/Dual Port RAM  ram_size=9
      settings: SourceProductBaseCode=SL
  input_storage_for_processing : hdlsllib/HDL RAMs/Dual Port RAM  ram_size=9
      settings: SourceProductBaseCode=SL
  read_from_storage_value : Outport
  current_value : Outport  Port=2
  read_from_porcessing_addr : Outport  Port=3
  wires:
  input_storage_for_processing/2 -> current_value/1
  input_storage_for_processing/1 -> Terminator6/1
  input_storage/2 -> read_from_storage_value/1
  input_storage/1 -> Terminator/1
  Delay1/1 -> input_storage_for_processing/4, read_from_porcessing_addr/1
  Compare To Constant/1 -> input_storage_for_processing/3
  InputState/1 -> Compare To Constant/1
  wr_en/1 -> input_storage/3
  wr_address/1 -> input_storage_for_processing/2, input_storage/2, Delay1/1
  wr_din/1 -> input_storage_for_processing/1, input_storage/1
  read address/1 -> input_storage/4

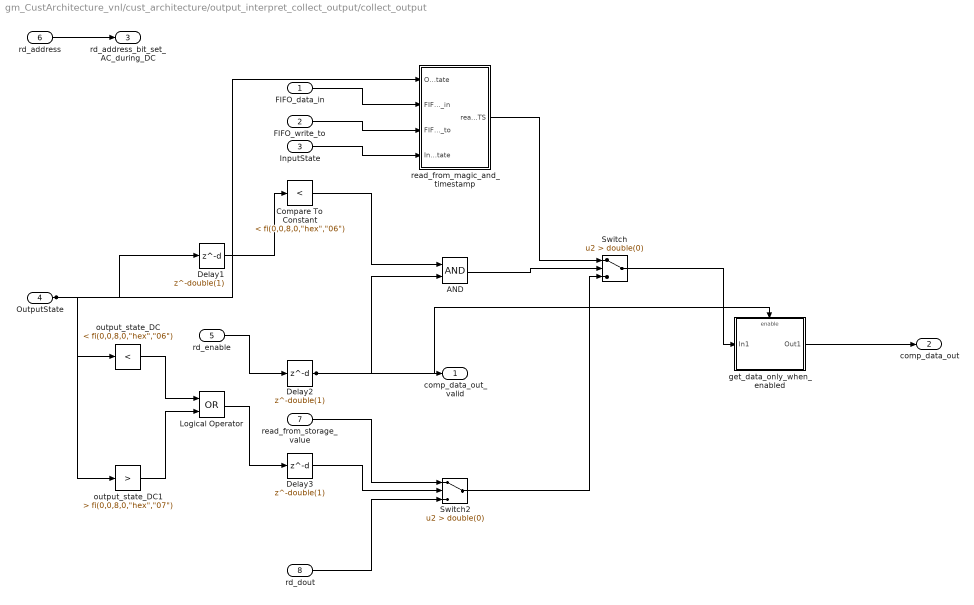
== system gm_CustArchitecture_vnl/cust_architecture/output_interpret_collect_output/collect_output ==
  FIFO_data_in : Inport  OutDataTypeStr=uint16  PortDimensions=1  SampleTime=1
  FIFO_write_to : Inport  Port=2  OutDataTypeStr=boolean  PortDimensions=1  SampleTime=1
  InputState : Inport  Port=3  OutDataTypeStr=uint8  PortDimensions=1  SampleTime=1
  OutputState : Inport  Port=4  OutDataTypeStr=uint8  PortDimensions=1  SampleTime=1
  rd_enable : Inport  Port=5  OutDataTypeStr=boolean  PortDimensions=1  SampleTime=1
  rd_address : Inport  Port=6  OutDataTypeStr=fixdt(0, 9, 0)  PortDimensions=1  SampleTime=1
  read_from_storage_value : Inport  Port=7  OutDataTypeStr=uint16  PortDimensions=1  SampleTime=1
  rd_dout : Inport  Port=8  OutDataTypeStr=uint16  PortDimensions=1  SampleTime=1
  AND : Logic  AllPortsSameDT=off  OutDataTypeStr=boolean  SampleTime=1
  Compare To Constant : simulink/Logic and Bit Operations/Compare To Constant  relop=<  const="fi(0,0,8,0,\"hex\",\"06\")"  OutDataTypeStr=boolean
  Delay1 : Delay  DelayLength=double(1)  InitialCondition=0  SampleTime=1
  Delay2 : Delay  DelayLength=double(1)  InitialCondition=0  SampleTime=1
  Delay3 : Delay  DelayLength=double(1)  InitialCondition=0  SampleTime=1
  Logical Operator : Logic  Operator=OR  AllPortsSameDT=off  OutDataTypeStr=boolean  SampleTime=1
  Switch : Switch  Criteria=u2 > Threshold  Threshold=double(0)  OutDataTypeStr=uint16  SampleTime=1
  Switch2 : Switch  Criteria=u2 > Threshold  Threshold=double(0)  OutDataTypeStr=uint16  SampleTime=1
  get_data_only_when_enabled : Subsystem
  output_state_DC : simulink/Logic and Bit Operations/Compare To Constant  relop=<  const="fi(0,0,8,0,\"hex\",\"06\")"  OutDataTypeStr=boolean
  output_state_DC1 : simulink/Logic and Bit Operations/Compare To Constant  relop=>  const="fi(0,0,8,0,\"hex\",\"07\")"  OutDataTypeStr=boolean
  read_from_magic_and_timestamp : Subsystem
  comp_data_out_valid : Outport
  comp_data_out : Outport  Port=2
  rd_address_bit_set_AC_during_DC : Outport  Port=3
  wires:
  read_from_magic_and_timestamp/1(read_from_Magic_TS) -> Switch/1
  output_state_DC1/1 -> Logical Operator/2
  output_state_DC/1 -> Logical Operator/1
  get_data_only_when_enabled/1(Out1) -> comp_data_out/1
  Switch2/1 -> Switch/3
  Switch/1 -> get_data_only_when_enabled/1(In1)
  Logical Operator/1 -> Delay3/1
  Delay3/1 -> Switch2/2
  Delay2/1 -> comp_data_out_valid/1, get_data_only_when_enabled/Enable, AND/2
  Delay1/1 -> Compare To Constant/1
  Compare To Constant/1 -> AND/1
  AND/1 -> Switch/2
  rd_dout/1 -> Switch2/3
  read_from_storage_value/1 -> Switch2/1
  rd_address/1 -> rd_address_bit_set_AC_during_DC/1
  rd_enable/1 -> Delay2/1
  OutputState/1 -> read_from_magic_and_timestamp/1(OutputState), Delay1/1, output_state_DC/1, output_state_DC1/1
  InputState/1 -> read_from_magic_and_timestamp/4(InputState)
  FIFO_write_to/1 -> read_from_magic_and_timestamp/3(FIFO_write_to)
  FIFO_data_in/1 -> read_from_magic_and_timestamp/2(FIFO_data_in)

== system gm_CustArchitecture_vnl/cust_architecture/output_interpret_collect_output/output_interpret ==
  data_stream_enable : Inport  OutDataTypeStr=uint8  PortDimensions=1  SampleTime=1
  InputState : Inport  Port=2  OutDataTypeStr=uint8  PortDimensions=1  SampleTime=1
  Interpret_to_RAM_output : Subsystem
  OutputStateMachine : Subsystem
  OutputState : Outport
  rd_enable : Outport  Port=2
  read_output_data_input_interpret_store_retrieve : Outport  Port=3
  wires:
  OutputStateMachine/1(OutputState) -> OutputState/1, Interpret_to_RAM_output/1(OutputState)
  Interpret_to_RAM_output/2(read address) -> read_output_data_input_interpret_store_retrieve/1
  Interpret_to_RAM_output/1(rd_enable) -> rd_enable/1
  InputState/1 -> OutputStateMachine/1(input_state)
  data_stream_enable/1 -> Interpret_to_RAM_output/2(data_stream_en)

== system gm_CustArchitecture_vnl/cust_architecture/spike_detection/LocalMaxima ==
  filter_output : Inport  OutDataTypeStr=uint16  SampleTime=1
  filter_writing_enable : Inport  Port=2  OutDataTypeStr=boolean  SampleTime=1
  filter_writing_address : Inport  Port=3  OutDataTypeStr=fixdt(0, 9, 0)  SampleTime=1
  Delay1 : Delay  DelayLength=1  InitialCondition=0
  Delay2 : Delay  DelayLength=1  InitialCondition=0
  Logical Operator1 : Logic  Inputs=3  IconShape=distinctive  AllPortsSameDT=off  OutDataTypeStr=boolean
  Terminator1 : Terminator
  Terminator2 : Terminator
  check_t-1 : RelationalOperator  Operator=<  OutDataTypeStr=boolean  RndMeth=Simplest
  check_t-2 : RelationalOperator  Operator=<  OutDataTypeStr=boolean  RndMeth=Simplest
  sample_t-1 : hdlsllib/HDL RAMs/Dual Port RAM  ram_size=9
      settings: SourceProductBaseCode=SL
  sample_t-2 : hdlsllib/HDL RAMs/Dual Port RAM  ram_size=9
      settings: SourceProductBaseCode=SL
  threshold : simulink/Logic and Bit Operations/Compare To Constant  relop=<  const=(th/(0.195))+32768  OutDataTypeStr=boolean
  detection_check : Outport
  wires:
  threshold/1 -> Logical Operator1/1
  sample_t-2/2 -> check_t-1/2
  sample_t-2/1 -> Terminator1/1
  sample_t-1/2 -> sample_t-2/1, check_t-1/1, check_t-2/1, threshold/1
  sample_t-1/1 -> Terminator2/1
  check_t-2/1 -> Logical Operator1/3
  check_t-1/1 -> Logical Operator1/2
  Logical Operator1/1 -> detection_check/1
  Delay2/1 -> sample_t-2/2
  Delay1/1 -> sample_t-1/2
  filter_writing_address/1 -> sample_t-2/4, sample_t-1/4, Delay1/1, Delay2/1
  filter_writing_enable/1 -> sample_t-2/3, sample_t-1/3
  filter_output/1 -> sample_t-1/1, check_t-2/2

== system gm_CustArchitecture_vnl/cust_architecture/spike_detection/refractory_period ==
  filter_writing_enable : Inport  OutDataTypeStr=boolean  SampleTime=1
  spike_check : Inport  Port=2  OutDataTypeStr=boolean  SampleTime=1
  filter_writing_address : Inport  Port=3  OutDataTypeStr=fixdt(0, 9, 0)  SampleTime=1
  read_filter_output_or_spike : Inport  Port=4  OutDataTypeStr=fixdt(0, 9, 0)  SampleTime=1
  Constant : Constant  OutDataTypeStr=uint16  SampleTime=-1
  Constant1 : Constant  Value=0  OutDataTypeStr=uint16  SampleTime=-1
  Delay : Delay  DelayLength=1  InitialCondition=0
  HDL Counter : hdlsllib/Sources/HDL Counter  CountType=Free running  CountInit=0  CountStep=1  CountMax=2^32  CountFromType=Initial value  CountFrom=0  CountResetPort=off  CountLoadPort=off  CountEnbPort=on  CountDirPort=off  CountDataType=Unsigned  CountWordLen=32  CountFracLen=0  CountSampTime=1
  Logical Operator : Logic  IconShape=distinctive  AllPortsSameDT=off  OutDataTypeStr=boolean
  Sum : Sum  Inputs=+-
  Switch : Switch  Criteria=u2 > Threshold
  Terminator2 : Terminator
  Terminator3 : Terminator
  rd_addr_check : simulink/Logic and Bit Operations/Compare To Constant  relop===  const=1  OutDataTypeStr=boolean
  refractory_period : simulink/Logic and Bit Operations/Compare To Constant  relop=>=  const=refractory  OutDataTypeStr=boolean
  spikes : hdlsllib/HDL RAMs/Dual Port RAM  ram_size=9
      settings: SourceProductBaseCode=SL
  timestamp_before : hdlsllib/HDL RAMs/Dual Port RAM  ram_size=9
      settings: SourceProductBaseCode=SL
  refractory_check : Outport
  spike : Outport  Port=2
  wires:
  timestamp_before/2 -> Sum/2
  timestamp_before/1 -> Terminator2/1
  spikes/2 -> spike/1
  spikes/1 -> Terminator3/1
  refractory_period/1 -> Logical Operator/1
  rd_addr_check/1 -> HDL Counter/1
  Switch/1 -> spikes/1
  Sum/1 -> refractory_period/1
  Logical Operator/1 -> refractory_check/1
  HDL Counter/1 -> timestamp_before/1, Sum/1
  Delay/1 -> timestamp_before/2, spikes/2
  Constant1/1 -> Switch/3
  Constant/1 -> Switch/1
  read_filter_output_or_spike/1 -> spikes/4, rd_addr_check/1
  filter_writing_address/1 -> timestamp_before/4, Delay/1
  spike_check/1 -> timestamp_before/3, Switch/2
  filter_writing_enable/1 -> spikes/3, Logical Operator/2

== system gm_CustArchitecture_vnl/cust_architecture/spike_detection/spike_check ==
  detection_check : Inport  OutDataTypeStr=boolean  SampleTime=1
  refractory_check : Inport  Port=2  OutDataTypeStr=boolean  SampleTime=1
  Logical Operator : Logic  AllPortsSameDT=off  OutDataTypeStr=boolean  SampleTime=1
  spike_check : Outport
  wires:
  Logical Operator/1 -> spike_check/1
  refractory_check/1 -> Logical Operator/2
  detection_check/1 -> Logical Operator/1

== system gm_CustArchitecture_vnl/cust_architecture/Butter_1st_HP/Subsystem/one_pole_IIR ==
  output_data_to_process : Inport  OutDataTypeStr=uint16  PortDimensions=1  SampleTime=1
  previous_sample : Inport  Port=2  OutDataTypeStr=fixdt(1, 16, -3)  PortDimensions=1  SampleTime=1
  Constant : Constant  Value=32768  OutDataTypeStr=fixdt(0,16,0)  SampleTime=-1
  Constant1 : Constant  Value=32768  OutDataTypeStr=fixdt(0,16,0)  SampleTime=-1
  HP_Butter_1st : Subsystem
  Subtract : Sum  Inputs=+-  OutDataTypeStr=fixdt(1,16,-3)
  Subtract1 : Sum  OutDataTypeStr=fixdt(0,16,0)
  filter_output : Outport  InitialOutput=[0]
  new_previous_sample : Outport  Port=2  InitialOutput=[0]
  wires:
  Subtract1/1 -> filter_output/1
  Subtract/1 -> HP_Butter_1st/1(Input2)
  HP_Butter_1st/2(Output1) -> new_previous_sample/1
  HP_Butter_1st/1(Output) -> Subtract1/1
  Constant1/1 -> Subtract1/2
  Constant/1 -> Subtract/2
  previous_sample/1 -> HP_Butter_1st/2(Input1)
  output_data_to_process/1 -> Subtract/1
